simulink model "NeuromuscularModelwReflex2"  (R2019b)
settings: Solver=ode15s  StartTime=0.0  StopTime=30  MaxStep=.01  RelTol=1e-4  AbsTol=1e-6  EnableMultiTasking=on
values from neighbouring files (symbols this model uses):
  dt_visual = 1/30    (= 0.0333333333333)    [evaluateCost.m]    (also in optimize.m)
  LceOffsetTA = 1-0.5*w    [ControlParams.m]
  legAngleTgt = 1.2    [ControlParams.m]    (also in assignGains_novirtmuscle.m = Gains(38))
  LlegLengthClr = .9    (= 0.9)    [ControlParams.m]    (also in assignGains.m = Gains(39); assignGains_novirtmuscle.m = Gains(20))
  LongDelay = 0.020    (= 0.02)    [ControlParams.m]
  MidDelay = 0.010    (= 0.01)    [ControlParams.m]
  RlegLengthClr = .9    (= 0.9)    [ControlParams.m]    (also in assignGains.m = Gains(83); assignGains_novirtmuscle.m = Gains(34))
  ShortDelay = 0.005    [ControlParams.m]
  simbiconGainD = 5*pi/180    (= 0.0872664625997)    [ControlParams.m]    (also in assignGains_novirtmuscle.m = Gains(35))
  simbiconGainV = 5*pi/180    (= 0.0872664625997)    [ControlParams.m]    (also in assignGains_novirtmuscle.m = Gains(36))
  simbiconLegAngle0 = 85*pi/180    (= 1.4835298642)    [ControlParams.m]    (also in assignGains_novirtmuscle.m = Gains(37))
  termination_height = 0.5    [ControlParams.m]
undefined symbols (not defined in the file or in its folder): footCenterToCGDist, footInertia, footMass, g, loptGAS, loptHAM, loptHAMCut, loptTA, lslackGAS, lslackHAM, lslackHAMCut, phimaxGASa, phimaxGASk, phimaxHAMk, phirefGASa, phirefGASk, phirefHAMh, phirefHAMk, rGASa, rGASk, rHAMh, rHAMk, rhoGASa, rhoGASk, rhoHAMh, rhoHAMk, X, Y, Z
libraries: NeuroMuscularLibrary x88, sm_lib x22, nesl_utility x20, simulink x6, simulink_extras x2
(part 1 of 3)
settings Model: ParamWorkspaceSource=ReferencedWorkspace  ExtModeTrigDuration=100  TunableVars=LGainGAS,LGainGLU,LGainHAM,LGainKneeOverExt,LGainSOL,LGainSOLTA,LGainTA,LGainVAS,LKglu,LPosGainGG,LSpeedGainGG,LhipDGain,LhipPGain,LkneeExtendGain,LkneeFlexGain,LkneeHoldGain1,LkneeHoldGain2,LkneeStopGain,LlegAngleFilter,LlegLengthClr,PsimbiconGainD,PsimbiconGainV,PsimbiconLegAngle0,RGainGAS,RGainGLU,RGainHAM,RGainHAMCut,RGainKneeOverExt,RGainSOL,RGainSOLTA,RGainTA,RGainVAS,RKglu,RPosGainGG,RSpeedGainGG,RhipDGain,RhipPGain,RkneeExtendGain,RkneeFlexGain,RkneeHoldGain1,RkneeHoldGain2,RkneeStopGain,RlegAngleFilter,RlegLengthClr,ankleDgain,ankleFilterPID,ankleFilterSEA,anklePgain,groundTheta,groundX,groundZ,impulseTime,impulseValue,kneeDgain,kneeFilterPID,kneeFilterSEA,kneePgain,legAngleTgt,simbiconGainD,simbiconGainV,simbiconLegAngle0  TunableVarsStorageClass=Auto,Auto,Auto,Auto,Auto,Auto,Auto,Auto,Auto,Auto,Auto,Auto,Auto,Auto,Auto,Auto,Auto,Auto,Auto,Auto,Auto,Auto,Auto,Auto,Auto,Auto,Auto,Auto,Auto,Auto,Auto,Auto,Auto,Auto,Auto,Auto,Auto,Auto,Auto,Auto,Auto,Auto,Auto,Auto,Auto,Auto,Auto,Auto,Auto,Auto,Auto,Auto,Auto,Auto,Auto,Auto,Auto,Auto,Auto,Auto,Auto  TunableVarsTypeQualifier=,,,,,,,,,,,,,,,,,,,,,,,,,,,,,,,,,,,,,,,,,,,,,,,,,,,,,,,,,,,,  Creator=nitisht  LastModifiedBy=Nathan
settings SolverCC: AutoScaleAbsTol=off  ZeroCrossAlgorithm=Adaptive
settings DataIOCC: LimitDataPoints=on  SaveFinalState=on  SaveFormat=StructureWithTime  SaveOutput=off  SaveState=on  ReturnWorkspaceOutputs=off  StateSaveName=tmp_raccel_xout  SignalLoggingName=tmp_raccel_logsout
settings OptimizationCC: DefaultParameterBehavior=Inlined  InlineInvariantSignals=on  EnhancedBackFolding=on  EfficientMapNaN2IntZero=off  LifeSpan=inf  SimCompilerOptimization=on  AccelVerboseBuild=on
settings DebuggingCC: AlgebraicLoopMsg=error  SaveWithDisabledLinksMsg=none  UnderspecifiedInitializationDetection=Classic  MergeDetectMultiDrivingBlocksExec=none  TimeAdjustmentMsg=warning  MaskedZcDiagnostic=none  IgnoredZcDiagnostic=none  SolverPrmCheckMsg=warning  StateNameClashWarn=warning  SFUnexpectedBacktrackingDiag=warning  SFNoUnconditionalDefaultTransitionDiag=warning  SFExecutionAtInitializationDiag=none  ArithmeticOperatorsInVariantConditions=warning
settings HardwareCC: ProdBitPerLong=64  ProdLargestAtomicFloat=None  ProdHWDeviceType=Intel->x86-64  TargetBitPerPointer=64  TargetBitPerSizeT=64  TargetBitPerPtrDiffT=64  TargetLongLongMode=on  TargetIntDivRoundTo=Zero  TargetEndianess=LittleEndian  TargetWordSize=64  TargetHWDeviceType=MATLAB Host  ProdEqTarget=off
settings ModelReferenceCC: UpdateModelReferenceTargets=IfOutOfDate  PropagateSignalLabelsOutOfModel=off
settings SFSimCC: SFSimEcho=off  SimUseLocalCustomCode=off  CustomCodeUndefinedFunction=UseInterfaceOnly
settings RTWCC: SystemTargetFile=raccel.tlc  TemplateMakefile=raccel_default_tmf  RTWUseLocalCustomCode=off  RTWUseSimCustomCode=on
settings CodeAppCC: GenerateComments=off  MaxIdLength=128  MangleLength=10  SimulinkBlockComments=off
settings RaccelTargetCC: GeneratePreprocessorConditionals=Disable all  MultiInstanceERTCode=off  PreserveStateflowLocalDataDimensions=off  ENABLE_SLEXEC_SSBRIDGE=0  RTWCAPIParams=off
settings ConfigComp: CovMetricSettings=dw  CovHtmlReporting=on  CovSaveCumulativeToWorkspaceVar=on  CovSaveSingleToWorkspaceVar=on  CovExternalEMLEnable=off  CovSFcnEnable=off
settings SimscapeCC: SimscapeNormalizeSystem=off
settings ConfigurationSet: Description=SimMechanics 2G
settings ExplorerConfigSet: InternalSimMechanicsExplorerSettings="<ExplorerConfiguration><canonicalview>default</canonicalview><AnimationSetting><BasePlaybackSpeed>1.0</BasePlaybackSpeed><PlaybackSpeedFactor>1.0</PlaybackSpeedFactor></AnimationSetting><TilePanel><TileInfo><Tiles Columns=\"1\" Count=\"1\" Rows=\"1\"><Column Weight=\"1\"/><Row Weight=\"1\"/><Tile Height=\"1\" Width=\"1\" X=\"0\" Y=\"0\"/></Tiles></TileInfo><SceneInfo><SceneViewer><BGColor><R>0.60000002384185791</R><G>0.60000002384185791</G><B>0.60000002384185791</B></BGColor><Camera><DoPerspective>on</DoPerspective><Position><X>39.4832183775192931</X><Y>-2.85000000000000187</Y><Z>0.960909521645701314</Z></Position><Center><X>39.4832183775192931</X><Y>-1.85000000000000187</Y><Z>0.960909521645701314</Z></Center><Up><X>0</X><Y>0</Y><Z>1</Z></Up><ViewLimDist>1</ViewLimDist><YLim>0.466307658154998583</YLim><XLim>0.868823709895729546</XLim></Camera></SceneViewer></SceneInfo></TilePanel><MechEditorPanel><Cameras><Camera><Id>Camera1</Id><Value><Name>Whole Body</Name><NativeCamera><PositionTrackingFeature>Prosthetic_Body_Mechanics_Layer.Whole_Body_Tracking_Camera.R</PositionTrackingFeature><CenterTrackingFeature>Prosthetic_Body_Mechanics_Layer.World_Frame_X_forward_Y_lateral_Z_up.W</CenterTrackingFeature><UpVectorTrackingFeature>Prosthetic_Body_Mechanics_Layer.World_Frame_X_forward_Y_lateral_Z_up.W</UpVectorTrackingFeature><CenterTrackingOrigin>off</CenterTrackingOrigin><CenterTrackingDirection>+Y</CenterTrackingDirection><UpVectorTrackingDirection>+Z</UpVectorTrackingDirection></NativeCamera></Value></Camera><Camera><Id>Camera2</Id><Value><Name>Prosthesis</Name><NativeCamera><PositionTrackingFeature>Prosthetic_Body_Mechanics_Layer.Prosthesis_Tracking_Camera.R</PositionTrackingFeature><CenterTrackingFeature>Prosthetic_Body_Mechanics_Layer.World_Frame_X_forward_Y_lateral_Z_up.W</CenterTrackingFeature><UpVectorTrackingFeature>Prosthetic_Body_Mechanics_Layer.World_Frame_X_forward_Y_lateral_Z_up.W</UpVectorTrackingFeature><CenterTrackingOrigin>off</CenterTrackingOrigin><CenterTrackingDirection>+Y</CenterTrackingDirection><UpVectorTrackingDirection>+Z</UpVectorTrackingDirection></NativeCamera></Value></Camera></Cameras><GfxPanelCameraMap><MapElement CameraMLId=\"Camera1\" GfxPanelIndex=\"0\"/></GfxPanelCameraMap><VideoCreator><PlaybackSpeedRatio>1</PlaybackSpeedRatio><FrameRate>30</FrameRate><VideoFormat>MPEG-4</VideoFormat><FrameSize>auto</FrameSize></VideoCreator></MechEditorPanel></ExplorerConfiguration>"

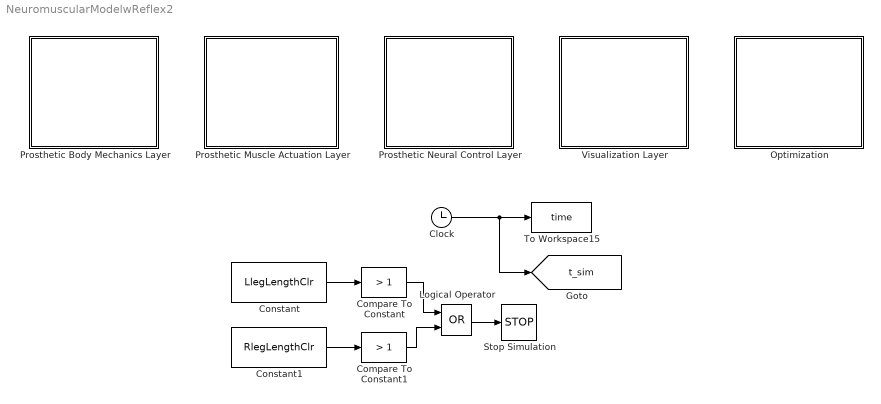
== system NeuromuscularModelwReflex2 ==
  Clock : Clock
  Compare To Constant : simulink/Logic and Bit Operations/Compare To Constant  relop=>  const=1  OutDataTypeStr=boolean
  Compare To Constant1 : simulink/Logic and Bit Operations/Compare To Constant  relop=>  const=1  OutDataTypeStr=boolean
  Constant : Constant  Value=LlegLengthClr
  Constant1 : Constant  Value=RlegLengthClr
  Logical Operator : Logic  Operator=OR  AllPortsSameDT=off  OutDataTypeStr=boolean
  Optimization : Subsystem
  Prosthetic Body Mechanics Layer : Subsystem
  Prosthetic Muscle Actuation Layer : Subsystem
  Prosthetic Neural Control Layer : Subsystem
  Stop Simulation : Stop
  To Workspace15 : ToWorkspace  VariableName=time  SampleTime=dt_visual
  Visualization Layer : Subsystem
  tag scope: t_sim=global
  wires:
  Clock/1 -> [t_sim], To Workspace15/1
  Compare To Constant/1 -> Logical Operator/1
  Logical Operator/1 -> Stop Simulation/1
  Compare To Constant1/1 -> Logical Operator/2
  Constant1/1 -> Compare To Constant1/1
  Constant/1 -> Compare To Constant/1

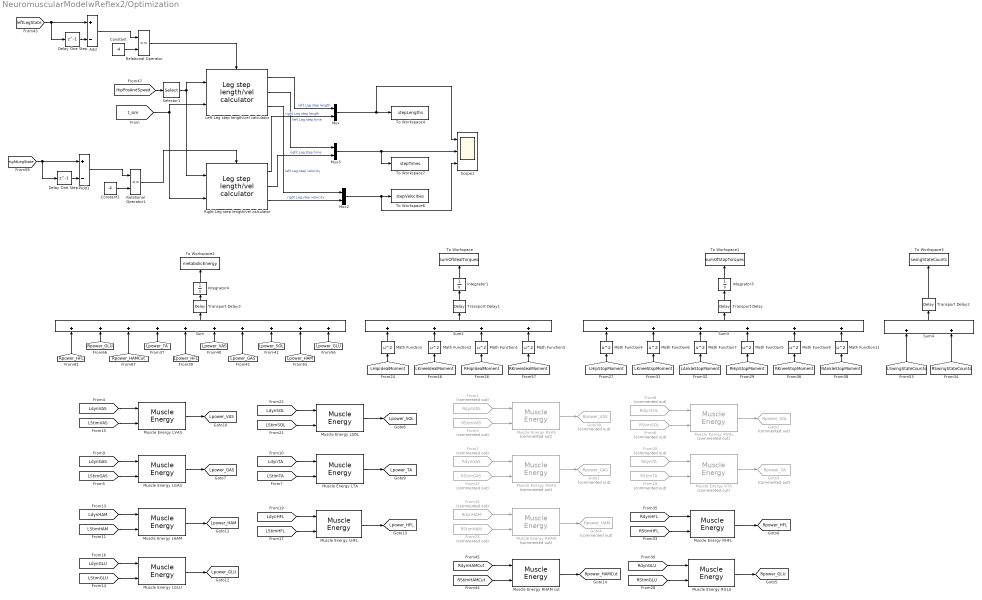
== system NeuromuscularModelwReflex2/Optimization ==
  Add : Sum  Inputs=+-
  Add1 : Sum  Inputs=+-
  Constant : Constant  Value=-4
  Constant1 : Constant  Value=-4
  Delay One Step : Delay  DelayLength=1
  Delay One Step1 : Delay  DelayLength=1
  From1 : From  Commented=on  GotoTag=RdynVAS  TagVisibility=global
  From12 : From  Commented=on  GotoTag=RStimGAS  TagVisibility=global
  From18 : From  Commented=on  GotoTag=RStimTA  TagVisibility=global
  From2 : From  Commented=on  GotoTag=RdynGAS  TagVisibility=global
  From20 : From  Commented=on  GotoTag=RdynTA  TagVisibility=global
  From23 : From  Commented=on  GotoTag=RStimHAM  TagVisibility=global
  From25 : From  Commented=on  GotoTag=RdynHAM  TagVisibility=global
  From3 : From  Commented=on  GotoTag=RStimVAS  TagVisibility=global
  From6 : From  Commented=on  GotoTag=RStimSOL  TagVisibility=global
  From8 : From  Commented=on  GotoTag=RdynSOL  TagVisibility=global
  Goto1 : Goto  Commented=on  GotoTag=Rpower_GAS  TagVisibility=global
  Goto2 : Goto  Commented=on  GotoTag=Rpower_SOL  TagVisibility=global
  Goto3 : Goto  Commented=on  GotoTag=Rpower_TA  TagVisibility=global
  Goto30 : Goto  Commented=on  GotoTag=Rpower_VAS  TagVisibility=global
  Goto4 : Goto  Commented=on  GotoTag=Rpower_HAM  TagVisibility=global
  Integrator1 : Integrator
  Integrator3 : Integrator
  Integrator4 : Integrator
  Left Leg step length/vel calculator : NeuroMuscularLibrary/Leg step length//vel calculator  SystemSampleTime=-1  Latency=0  AutoFrameSizeCalculation=off
  Math Function{,1..7,9,11} (10 alike) : Math  Operator=square  SaturateOnIntegerOverflow=on
  Muscle Energy LGAS : NeuroMuscularLibrary/Muscle Energy  lopt=loptGAS  FT=FT_GAS  Fmax=FmaxGAS  vmax=vmaxGLU
  Muscle Energy LGLU : NeuroMuscularLibrary/Muscle Energy  lopt=loptGLU  FT=FT_GLU  Fmax=FmaxGLU  vmax=vmaxGLU
  Muscle Energy LHAM : NeuroMuscularLibrary/Muscle Energy  lopt=loptHAM  FT=FT_HAM  Fmax=FmaxHAM  vmax=vmaxGLU
  Muscle Energy LHFL : NeuroMuscularLibrary/Muscle Energy  lopt=loptHFL  FT=FT_HFL  Fmax=FmaxHFL  vmax=vmaxGLU
  Muscle Energy LSOL : NeuroMuscularLibrary/Muscle Energy  lopt=loptSOL  FT=FT_SOL  Fmax=FmaxSOL  vmax=vmaxGLU
  Muscle Energy LTA : NeuroMuscularLibrary/Muscle Energy  lopt=loptTA  FT=FT_TA  Fmax=FmaxTA  vmax=vmaxGLU
  Muscle Energy LVAS : NeuroMuscularLibrary/Muscle Energy  lopt=loptVAS  FT=FT_VAS  Fmax=FmaxVAS  vmax=vmaxGLU
  Muscle Energy RGAS : NeuroMuscularLibrary/Muscle Energy  Commented=on  lopt=loptGAS  FT=FT_GAS  Fmax=FmaxGAS  vmax=vmaxGLU
  Muscle Energy RGLU : NeuroMuscularLibrary/Muscle Energy  lopt=loptGLU  FT=FT_GLU  Fmax=FmaxGLU  vmax=vmaxGLU
  Muscle Energy RHAM : NeuroMuscularLibrary/Muscle Energy  Commented=on  lopt=loptHAM  FT=FT_HAM  Fmax=FmaxHAM  vmax=vmaxGLU
  Muscle Energy RHAM cut : NeuroMuscularLibrary/Muscle Energy  lopt=loptHAMCut  FT=FT_HAM  Fmax=FmaxHAMCut  vmax=vmaxGLU
  Muscle Energy RHFL : NeuroMuscularLibrary/Muscle Energy  lopt=loptHFL  FT=FT_HFL  Fmax=FmaxHFL  vmax=vmaxGLU
  Muscle Energy RSOL : NeuroMuscularLibrary/Muscle Energy  Commented=on  lopt=loptSOL  FT=FT_SOL  Fmax=FmaxSOL  vmax=vmaxGLU
  Muscle Energy RTA : NeuroMuscularLibrary/Muscle Energy  Commented=on  lopt=loptTA  FT=FT_TA  Fmax=FmaxTA  vmax=vmaxGLU
  Muscle Energy RVAS : NeuroMuscularLibrary/Muscle Energy  Commented=on  lopt=loptVAS  FT=FT_VAS  Fmax=FmaxVAS  vmax=vmaxGLU
  Mux : Mux  Inputs=2
  Mux2 : Mux  Inputs=2
  Mux3 : Mux  Inputs=2
  Relational Operator : RelationalOperator  Operator=<=  OutDataTypeStr=boolean  RndMeth=Simplest
  Relational Operator1 : RelationalOperator  Operator=<=  OutDataTypeStr=boolean  RndMeth=Simplest
  Right Leg step length/vel calculator : NeuroMuscularLibrary/Leg step length//vel calculator  SystemSampleTime=-1  Latency=0  AutoFrameSizeCalculation=off
  Scope1 : Scope  NumInputPorts=3
  Selector1 : Selector  InputPortWidth=3  IndexOptions=Index vector (dialog)  Indices=[1]  OutputSizes=1
  Sum : Sum  Inputs=++++++++++
  Sum2 : Sum  Inputs=++++
  Sum3 : Sum  Inputs=++++++
  Sum4 : Sum
  To Workspace : ToWorkspace  VariableName=sumOfIdealTorques  SampleTime=-1
      settings: MaxDataPoints=1
  To Workspace1 : ToWorkspace  VariableName=sumOfStopTorques  SampleTime=-1
      settings: MaxDataPoints=1
  To Workspace2 : ToWorkspace  VariableName=metabolicEnergy  SampleTime=-1
      settings: MaxDataPoints=1
  To Workspace3 : ToWorkspace  VariableName=swingStateCounts  SampleTime=-1
      settings: MaxDataPoints=1
  To Workspace4 : ToWorkspace  VariableName=stepLengths  SampleTime=-1
  To Workspace6 : ToWorkspace  VariableName=stepVelocities  SampleTime=-1
  To Workspace7 : ToWorkspace  VariableName=stepTimes  SampleTime=-1
  Transport Delay{,1..3} (4 alike) : TransportDelay  DelayTime=3  BufferSize=24576
  tag scope: Lpower_GAS=global, Lpower_GLU=global, Lpower_HAM=global, Lpower_HFL=global, Lpower_SOL=global, Lpower_TA=global, Lpower_VAS=global, Rpower_GLU=global, Rpower_HAMCut=global, Rpower_HFL=global
  wires:
  Math Function5/1 -> Sum3/4
  Transport Delay1/1 -> Integrator1/1
  Sum2/1 -> Transport Delay1/1
  Transport Delay3/1 -> Integrator4/1
  Sum/1 -> Transport Delay3/1
  Integrator4/1 -> To Workspace2/1
  [Lpower_GAS] -> Sum/7
  [Lpower_SOL] -> Sum/8
  [Lpower_HAM] -> Sum/9
  [Lpower_GLU] -> Sum/10
  [Rpower_HAMCut] -> Sum/3
  [Lpower_TA] -> Sum/4
  [Lpower_HFL] -> Sum/5
  [Lpower_VAS] -> Sum/6
  [Rpower_GLU] -> Sum/2
  [Rpower_HFL] -> Sum/1
  [RSwingStateCounts] -> Sum4/2
  [LSwingStateCounts] -> Sum4/1
  Transport Delay2/1 -> To Workspace3/1
  Sum4/1 -> Transport Delay2/1
  Math Function11/1 -> Sum3/6
  [RAnkleStopMoment] -> Math Function11/1
  Math Function9/1 -> Sum3/5
  [RKneeStopMoment] -> Math Function9/1
  Transport Delay/1 -> Integrator3/1
  Sum3/1 -> Transport Delay/1
  [LAnkleStopMoment] -> Math Function7/1
  Math Function7/1 -> Sum3/3
  [RHipStopMoment] -> Math Function5/1
  [LKneeStopMoment] -> Math Function6/1
  Math Function6/1 -> Sum3/2
  [LHipStopMoment] -> Math Function4/1
  Math Function4/1 -> Sum3/1
  Integrator3/1 -> To Workspace1/1
  Math Function3/1 -> Sum2/4
  [RKneeIdealMoment] -> Math Function3/1
  Math Function1/1 -> Sum2/3
  [RHipIdealMoment] -> Math Function1/1
  [LKneeIdealMoment] -> Math Function2/1
  Math Function2/1 -> Sum2/2
  [LHipIdealMoment] -> Math Function/1
  Math Function/1 -> Sum2/1
  Integrator1/1 -> To Workspace/1
  Muscle Energy RHAM cut/1 -> [Rpower_HAMCut]
  [RStimHAMCut] -> Muscle Energy RHAM cut/2
  [RdynHAMCut] -> Muscle Energy RHAM cut/1
  [LdynVAS] -> Muscle Energy LVAS/1
  [LdynGAS] -> Muscle Energy LGAS/1
  Muscle Energy LHFL/1 -> [Lpower_HFL]
  Muscle Energy LGLU/1 -> [Lpower_GLU]
  Muscle Energy LHAM/1 -> [Lpower_HAM]
  [LStimHFL] -> Muscle Energy LHFL/2
  [LdynHFL] -> Muscle Energy LHFL/1
  [LStimGLU] -> Muscle Energy LGLU/2
  [LdynGLU] -> Muscle Energy LGLU/1
  [LStimHAM] -> Muscle Energy LHAM/2
  [LdynHAM] -> Muscle Energy LHAM/1
  [LStimTA] -> Muscle Energy LTA/2
  [LdynTA] -> Muscle Energy LTA/1
  Muscle Energy LTA/1 -> [Lpower_TA]
  Muscle Energy LSOL/1 -> [Lpower_SOL]
  Muscle Energy LGAS/1 -> [Lpower_GAS]
  Muscle Energy LVAS/1 -> [Lpower_VAS]
  [LStimGAS] -> Muscle Energy LGAS/2
  [LStimVAS] -> Muscle Energy LVAS/2
  [LStimSOL] -> Muscle Energy LSOL/2
  [LdynSOL] -> Muscle Energy LSOL/1
  From1/1 -> Muscle Energy RVAS/1
  From2/1 -> Muscle Energy RGAS/1
  Muscle Energy RHFL/1 -> [Rpower_HFL]
  Muscle Energy RGLU/1 -> [Rpower_GLU]
  Muscle Energy RHAM/1 -> Goto4/1
  [RStimHFL] -> Muscle Energy RHFL/2
  [RdynHFL] -> Muscle Energy RHFL/1
  [RStimGLU] -> Muscle Energy RGLU/2
  [RdynGLU] -> Muscle Energy RGLU/1
  From23/1 -> Muscle Energy RHAM/2
  From25/1 -> Muscle Energy RHAM/1
  From18/1 -> Muscle Energy RTA/2
  From20/1 -> Muscle Energy RTA/1
  Muscle Energy RTA/1 -> Goto3/1
  Muscle Energy RSOL/1 -> Goto2/1
  Muscle Energy RGAS/1 -> Goto1/1
  Muscle Energy RVAS/1 -> Goto30/1
  From12/1 -> Muscle Energy RGAS/2
  From3/1 -> Muscle Energy RVAS/2
  From6/1 -> Muscle Energy RSOL/2
  From8/1 -> Muscle Energy RSOL/1
  Mux3/1 -> Scope1/2, To Workspace7/1
  Right Leg step length/vel calculator/2 -> Mux3/2  "right Leg step time"
  Right Leg step length/vel calculator/3 -> Mux2/2  "right Leg step velocity"
  Left Leg step length/vel calculator/2 -> Mux3/1  "left Leg step time"
  [t_sim] -> Right Leg step length/vel calculator/2, Left Leg step length/vel calculator/2
  Left Leg step length/vel calculator/3 -> Mux2/1  "left Leg step velocity"
  Mux2/1 -> To Workspace6/1, Scope1/3
  Add1/1 -> Relational Operator1/1
  [leftLegState] -> Add/1, Delay One Step/1
  Delay One Step1/1 -> Add1/2
  Mux/1 -> To Workspace4/1, Scope1/1
  [rightLegState] -> Delay One Step1/1, Add1/1
  Relational Operator1/1 -> Right Leg step length/vel calculator/Enable
  Constant1/1 -> Relational Operator1/2
  Add/1 -> Relational Operator/1
  Delay One Step/1 -> Add/2
  Relational Operator/1 -> Left Leg step length/vel calculator/Enable
  Constant/1 -> Relational Operator/2
  Selector1/1 -> Right Leg step length/vel calculator/1, Left Leg step length/vel calculator/1
  Left Leg step length/vel calculator/1 -> Mux/1  "left Leg step length"
  [HipPosAndSpeed] -> Selector1/1
  Right Leg step length/vel calculator/1 -> Mux/2  "right Leg step length"
